simulink model "phdMain"  (R2023b)
settings: Solver=ode4  StartTime=0.0  StopTime=t.Data(end)  FixedStep=1e-3  RelTol=1e-3
undefined symbols (not defined in the file): A_bar, AEFF, B_E, C_bar, C_T, Cd_neg, Cd_pos, DiscIntNeverNeededParam, Gamma, H, k, K, L_gain, L_STROKE, M, m3PsToLpm, P_return_Pa, P_supply_Pa, PA_Pa, PaToBar, PB_Pa, Q, R, RHO, Ts, V01, V02, V_DEAD, v_mPs, W, xc_dot, xc_m
libraries: simulink x1
(part 3 of 3)

== matlab function phdMain/Nguyen Observer/Nguyen_Observer/phi_calc/MATLAB Function4 ==
  data: v input; F_stribeck output
function F_stribeck = fcn(v)


% close all 

% --- Geçiş Yumuşaklığı Parametresi ---
% Bu değer büyüdükçe 0'daki eğim azalır (daha eğimli geçer)
eps_smooth = 0.0223;
% eps_smooth = 0.015;

%%%
kv_p = 12; Fc_p = 25; Fs_p  = 383; tau_p = 0.016;
kv_n = 35; Fc_n = 7.5; Fs_n = 183; tau_n = 0.02016;
%%%


% Yumuşatılmış yön fonksiyonu (sign yerine tanh)
% Bu fonksiyon -1 ile 1 arasında yumuşak bir geçiş sağlar
smooth_sign = tanh(v ./ eps_smooth);

% Asimetrik katsayı vektörleri oluşturma
% Hızın yönüne göre katsayıları seçiyoruz
kv = (v >= 0)*kv_p + (v < 0)*kv_n;
Fc = (v >= 0)*Fc_p + (v < 0)*Fc_n;
Fs = (v >= 0)*Fs_p + (v < 0)*Fs_n;
tau = (v >= 0)*tau_p + (v < 0)*tau_n;
F_stribeck = (Fc .* smooth_sign) + (Fs .* smooth_sign .* exp(-abs(v./tau)));

== matlab function phdMain/SDRE_OBS_SNR/Subsystem/MATLAB Function1 ==
  data: Q1_calc input; Q2_calc input; x1_hat input; B_x output
function B_x = B_x(Q1_calc, Q2_calc, x1_hat)
D_PISTON    = 34e-3;                    % Piston Diameter m
D_ROD       = 30e-3;                    % Rod Diameter m
A_PISTON    = (pi * D_PISTON^2)/4;      % Piston area m^2
A_ROD       = (pi * D_ROD^2)/4;         % Rod area m^2
AEFF        = A_PISTON - A_ROD;         % Effective Area m2
L_STROKE    = 190.16e-3;                % Total Stroke Length m
V01         = AEFF * (L_STROKE/2);      % Initial Chamber Volume in neural position m^3
V02         = AEFF * (L_STROKE/2);      % Initial Chamber Volume in neural position m^3
V_DEAD      = 1.5315e-05;               % 15.3 cm^3 dead volume <- 
V0 = V01 + V_DEAD;                      % Total Volume m3

eps = 1e-6;                             % Epsilon for numerical stability 
%%
A_c = AEFF; 
V_0 = V0; 
beta = 1.6e9; 
%%

delta_1 = beta / ((V_0 + A_c*x1_hat ));
delta_2 = beta / ((V_0 - A_c*x1_hat ));


B_x =   [0; 
             0;
             delta_1 * Q1_calc;
             delta_2 * Q2_calc];% u>=0 ise,

end

== matlab function phdMain/SDRE_OBS_SNR/Subsystem/MATLAB Function2 ==
  data: u input; Q1 output; Ps input; Pr input; x3_hat input; x4_hat input; Q2 output; QR output
function [Q1, Q2, QR] = Q_fcn(u, Ps, Pr, x3_hat, x4_hat)

K_sv           = 0.00000334; 
k_sv           = 1.82709080;
    % x0 parametresini girişten kaldırdık, içeride asimetrik tanımlayacağız.
    
    % --- ASİMETRİK SIZINTI AYARLARI ---
    % Hedef: P_null = 70 bar (Ps=210 bar iken)
    % Bu dengeyi sağlamak için Return tarafı açıklığı daha büyük olmalı.

    % --- GÜNCELLENMİŞ ASİMETRİK SIZINTI AYARLARI ---
    % Hedef: Ps=200 bar, Pr=4.5 bar iken yaklaşık 70-75 bar denge basıncı
    % $$x_{0S} \cdot \sqrt{130} = x_{0R} \cdot \sqrt{70}$$ --> Ortalamaları
    % da bulunan x0 olacak.

    % Ortalama x0 = 0.53e-3 idi. Bunu asimetrik dağıtıyoruz:
    % x0_S = 0.47e-3;  % Supply tarafı (0.47 mA)
    % x0_R = 0.64e-3;  % Return tarafı (0.64 mA)
    
    x0_S = 0.46e-3 ;  % Supply tarafı (0.46 mA) --> bunu editledim
    x0_R = 0.64e-3 ;  % Return tarafı (0.64 mA)

    % x0_S = 0.53e-3;  % Supply tarafı (0.47 mA)
    % x0_R = 0.53e-3;  % Return tarafı (0.64 mA)

    K_tare = 2.345e-9; 
    
    % Güvenlik (Basınçlar)
    dPs1 = max(0, Ps - x3_hat); dP1r = max(0, x3_hat - Pr);
    dPs2 = max(0, Ps - x4_hat); dP2r = max(0, x4_hat - Pr);
    dPsr = max(0, Ps - Pr);

    if u >= 0
        % P_S -> P_1 (Supply Side - Ana Akış) -> x0_S kullan
        Q1_S = K_sv * sqrt(dPs1) * (x0_S + u); 
        
        % P_1 -> P_R (Return Side - Sızıntı) -> x0_R kullan
        Q1_R = K_sv * sqrt(dP1r) * (x0_R^2 / (x0_R + k_sv*u)); 

        % P_S -> P_2 (Supply Side - Sızıntı) -> x0_S kullan
        Q2_S = K_sv * sqrt(dPs2) * (x0_S^2 / (x0_S + k_sv*u)); 
        
        % P_2 -> P_R (Return Side - Ana Akış) -> x0_R kullan
        Q2_R = K_sv * sqrt(dP2r) * (x0_R + u);
    else
        % x < 0 durumu
        % Simetriyi korumak için x negatifken de Supply/Return rollerine göre
        % doğru x0'ı seçmeliyiz.
        
        % P_S -> P_1 (Supply Side - Sızıntı)
        Q1_S = K_sv * sqrt(dPs1) * (x0_S^2 / (x0_S - k_sv*u)); 
        
        % P_1 -> P_R (Return Side - Ana Akış)
        Q1_R = K_sv * sqrt(dP1r) * (x0_R - u); 

        % P_S -> P_2 (Supply Side - Ana Akış)
        Q2_S = K_sv * sqrt(dPs2) * (x0_S - u); 
        
        % P_2 -> P_R (Return Side - Sızıntı)
        Q2_R = K_sv * sqrt(dP2r) * (x0_R^2 / (x0_R - k_sv*u)); 
    end

    Q1 = Q1_S - Q1_R;
    Q2 = Q2_S - Q2_R;
    QR = Q1_R + (Q2_R) + K_tare * sqrt(dPsr); 
end

== matlab function phdMain/SDRE_Observer ==
  settings: updateMethod=DISCRETE  sampleTime=1e-3
  data: u_k input; dxhat output; z_k input; Ps input; Pr input; x_hat input; dP_flat output; P_flat input; x_hat_out output
function [dxhat, dP_flat, x_hat_out] = sdre_observer_ode(u_k, z_k, Ps, Pr, x_hat, P_flat)
% Port sırası:
%   Girişler:  1:u_k(1)  2:z_k(3)  3:Ps(1)  4:Pr(1)  5:x_hat(4)  6:P_flat(16)
%   Çıkışlar:  1:dxhat(4)  2:dP_flat(16)  3:x_hat_out(4)
%
% Integrator 1 → x_hat  (4×1),  IC = [0;0;0;0]
% Integrator 2 → P_flat (16×1), IC = P0(:)  where P0=diag([1e-4,1,1e5,1e5])

    %% Boyut zorlama
    x_hat  = x_hat(:);    % 4×1
    P_flat = P_flat(:);   % 16×1
    z_k    = z_k(:);      % 3×1

    %% Sistem Parametreleri
    m_p    = 3.4;
    D_P    = 34e-3;  D_R = 30e-3;
    A_c    = pi * (D_P^2 - D_R^2) / 4;
    L_S    = 190.16e-3;
    V_DEAD = 1.5315e-5;
    V_0    = A_c * (L_S / 2) + V_DEAD;
    C_t    = 3.9933e-13;
    beta   = 1.6e9;
    K_sv   = 3.34e-6;
    k_sv   = 1.82709080;

    %% Gözlemci Matrisleri
    Q_proc = diag([1e-3, 1e-2, 5e8, 5e8]);
    R_inv  = diag([1.0e7, 1.0e-2, 1.0e-2]);
    H      = [1 0 0 0;
              0 0 1 0;
              0 0 0 1];

    %% P matrisini yeniden oluştur
    P  = reshape(P_flat, 4, 4);

    x1 = x_hat(1);  x2 = x_hat(2);
    x3 = x_hat(3);  x4 = x_hat(4);

    %% Durum Bağımlı Matrisler
    A_k = local_A(x1, x2, beta, V_0, A_c, C_t, m_p);
    [Q1, Q2] = local_Q(u_k, Ps, Pr, x3, x4, K_sv, k_sv);
    f_k = local_B(x1, beta, V_0, A_c, Q1, Q2);

    %% Kalman Kazancı
    PHt = P * H';
    K   = PHt * R_inv;

    %% Gözlemci türevi
    dxhat = A_k * x_hat + f_k + K * (z_k - H * x_hat);

    %% Diferansiyel Riccati
    dP      = A_k*P + P*A_k' - PHt*R_inv*(H*P) + Q_proc;
    dP_flat = dP(:);

    x_hat_out = x_hat;
end

%% ---- Yerel Fonksiyonlar ----
function A_x = local_A(x1, x2, beta, V0, Ac, Ct, m)
    eps_v = 1e-6;
    if x2 >= 0
        Fc=6.93;   Fs=93.02;  tau_f=0.0357;  B=33.96;
    else
        Fc=19.39;  Fs=83.58;  tau_f=0.0382;  B=31.98;
    end
    Ff = tanh(x2)*(Fc + (Fs-Fc)*exp(-abs(x2)/tau_f));
    d1 = beta/(V0 + Ac*x1);
    d2 = beta/(V0 - Ac*x1);
    A_x = [0   1                             0        0    ;
           0  -B/m - Ff/(m*abs(x2)+eps_v)   Ac/m    -Ac/m ;
           0  -d1*Ac                        -d1*Ct    d1*Ct;
           0   d2*Ac                         d2*Ct   -d2*Ct];
end

function [Q1, Q2] = local_Q(x, Ps, Pr, P1, P2, K, k)
    x0S=0.46e-3;  x0R=0.64e-3;
    dPs1=max(0.0,Ps-P1);  dP1r=max(0.0,P1-Pr);
    dPs2=max(0.0,Ps-P2);  dP2r=max(0.0,P2-Pr);
    if x >= 0
        Q1 = K*sqrt(dPs1)*(x0S+x)           - K*sqrt(dP1r)*(x0R^2/(x0R+k*x));
        Q2 = K*sqrt(dPs2)*(x0S^2/(x0S+k*x)) - K*sqrt(dP2r)*(x0R+x);
    else
        Q1 = K*sqrt(dPs1)*(x0S^2/(x0S-k*x)) - K*sqrt(dP1r)*(x0R-x);
        Q2 = K*sqrt(dPs2)*(x0S-x)            - K*sqrt(dP2r)*(x0R^2/(x0R-k*x));
    end
end

function Bv = local_B(x1, beta, V0, Ac, Q1, Q2)
    Vd = 1.5315e-5;
    d1 = beta/(V0+Ac*x1+Vd);
    d2 = beta/(V0-Ac*x1+Vd);
    Bv = [0; 0; d1*Q1; d2*Q2];
end

== matlab function phdMain/SDRE_OBS_SNR/MATLAB Function3 ==
  data: x_1_hat input; A_k output; x_2_hat input
function A_k = A_k_discrete(x_1_hat, x_2_hat)
M           = 3.4;                      % Movable mass (Piston + Rod) kg
D_PISTON    = 34e-3;                    % Piston Diameter m
D_ROD       = 30e-3;                    % Rod Diameter m
A_PISTON    = (pi * D_PISTON^2)/4;      % Piston area m^2
A_ROD       = (pi * D_ROD^2)/4;         % Rod area m^2
AEFF        = A_PISTON - A_ROD;         % Effective Area m2
L_STROKE    = 190.16e-3;                % Total Stroke Length m
V01         = AEFF * (L_STROKE/2);      % Initial Chamber Volume in neural position m^3
V02         = AEFF * (L_STROKE/2);      % Initial Chamber Volume in neural position m^3
V_DEAD      = 1.5315e-05;               % 15.3 cm^3 dead volume 
V0          = V01 + V_DEAD;             % Total Volume m3
C_T         = 3.9933e-13;               % Internal leakage constant m3/s/Pa
eps_val     = 1e-6;                     % Epsilon for numerical stability 

%% Parametre Atamaları
m = M; 
C_t = C_T; 
A_c = AEFF; 
V_0 = V0; 
beta = 1.6e9; 
Ts = 1e-3; 
%% Sürtünme Dinamikleri ve Sönüm Katsayısı
if x_2_hat >= 0 
    F_c = 6.93; 
    F_s = 93.02; 
    tau = 0.0357; 
    B = 33.96; 
else 
    F_c = 19.39; 
    F_s = 83.58; 
    tau = 0.0382; 
    B = 31.98; 
end 

% Sürtünme denkleminde sign yerine tanh kullanımı (Sürekli türevlenebilirlik için)
F_frc = tanh(x_2_hat) * (F_c + (F_s - F_c) * exp(-abs(x_2_hat) / tau)); 

%% Matris Elemanlarının Hesaplanması (Sürekli Zaman Ac)
delta_1 = beta / (V_0 + A_c * x_1_hat);
delta_2 = beta / (V_0 - A_c * x_1_hat);

a22 = -B/m - F_frc / (m * abs(x_2_hat) + eps_val);
a23 = A_c/m;
a24 = -A_c/m;
a32 = -delta_1 * A_c; 
a33 = -delta_1 * C_t;
a34 = delta_1 * C_t;
a42 = delta_2 * A_c;
a43 = delta_2 * C_t;
a44 = -delta_2 * C_t;

% Sürekli Zaman Durum Matrisi
A_c_mat = [0    1       0       0; 
           0    a22     a23     a24; 
           0    a32     a33     a34; 
           0    a42     a43     a44];

%% Tustin Yöntemi ile Ayrıklaştırma (Discrete Time Ak)
I = eye(4);
% (I - 0.5*Ts*Ac)^-1 * (I + 0.5*Ts*Ac) işlemi sayısal verimlilik için mldivide (\) ile çözülür
A_k = (I - 0.5 * Ts * A_c_mat) \ (I + 0.5 * Ts * A_c_mat);

end

== matlab function phdMain/SDRE_OBS_SNR/MATLAB Function4 ==
  data: Q1_calc input; Q2_calc input; x1_hat input; B_k output; A_k input
function B_k = B_k_discrete(Q1_calc, Q2_calc, x1_hat, A_k)
    % Fiziksel Parametreler
    D_PISTON    = 34e-3;                    % Piston Diameter m
    D_ROD       = 30e-3;                    % Rod Diameter m
    A_PISTON    = (pi * D_PISTON^2)/4;      % Piston area m^2
    A_ROD       = (pi * D_ROD^2)/4;         % Rod area m^2
    AEFF        = A_PISTON - A_ROD;         % Effective Area m2
    L_STROKE    = 190.16e-3;                % Total Stroke Length m
    V01         = AEFF * (L_STROKE/2);      % Initial Chamber Volume m^3
    V_DEAD      = 1.5315e-05;               % 15.3 cm^3 dead volume 
    V0          = V01 + V_DEAD;             % Total Volume m3
    
    A_eff_area  = AEFF; 
    beta        = 1.6e9; 
    Ts = 1e-3; 
    
    % Sürekli Zaman B_c Vektörünün Hesaplanması
    delta_1 = beta / (V0 + A_eff_area * x1_hat);
    delta_2 = beta / (V0 - A_eff_area * x1_hat);
    
    B_c = [0; 
           0;
           delta_1 * Q1_calc;
           delta_2 * Q2_calc];
           
    % Tustin cebirsel dönüşümü ile Ak entegrasyonu
    I = eye(4);
    B_k = (Ts / 2) * (I + A_k) * B_c;
end

== matlab function phdMain/SDRE_OBS_SNR/MATLAB Function5 ==
  data: x_hat input; A_k output; u_k input; B_k output; Ps_k input; Pr_k input
function [A_k, B_k] = discrete_system_matrices(x_hat, u_k, Ps_k, Pr_k)
    % 1. Sistem Geometrisi ve Tanımlamalar
    x1_hat = x_hat(1); 
    x2_hat = x_hat(2); 
    x3_hat = x_hat(3); 
    x4_hat = x_hat(4); 
    
    M           = 3.4;
    D_PISTON    = 34e-3;
    D_ROD       = 30e-3;
    A_eff_area  = (pi * D_PISTON^2)/4 - (pi * D_ROD^2)/4;
    L_STROKE    = 190.16e-3;
    V0          = A_eff_area * (L_STROKE/2) + 1.5315e-05;
    C_t         = 3.9933e-13;
    eps_val     = 1e-6;
    B_E = 1.6e9;
%%
    % 2. Sürtünme ve Diferansiyel Değişkenler
    if x2_hat >= 0 
        F_c = 6.93; F_s = 93.02; tau = 0.0357; B = 33.96; 
    else 
        F_c = 19.39; F_s = 83.58; tau = 0.0382; B = 31.98; 
    end 

    F_frc = tanh(x2_hat) * (F_c + (F_s - F_c) * exp(-(abs(x2_hat)^2) / tau^2)); 
    
    delta_1 = B_E / (V0 + A_eff_area * x1_hat + eps_val);
    delta_2 = B_E / (V0 - A_eff_area * x1_hat + eps_val);

    % 3. Sürekli Zaman Ac Matris Elemanları
    a22 = -B/M - F_frc / ((M * x2_hat) + eps_val);

    a23 = A_eff_area/M;  a24 = -A_eff_area/M;
    a32 = -delta_1 * A_eff_area; 
    a33 = -delta_1 * C_t; 
    a34 = delta_1 * C_t;
    a42 = delta_2 * A_eff_area;  
    a43 = delta_2 * C_t;  
    a44 = -delta_2 * C_t;

    A_c_mat = [0    1       0       0; 
               0    a22     a23     a24; 
               0    a32     a33     a34; 
               0    a42     a43     a44];
    

      % Valf Parametreleri
    K_sv = 0.00000334; 
    k_sv = 1.82709080;
    K_tare = 2.345e-9; 
    
    % Asimetrik Sızıntı Ayarları (Sıfır Geçiş Dengesi)
    x0_S = 0.46e-3;  % Supply tarafı (0.46 mA)
    x0_R = 0.64e-3;  % Return tarafı (0.64 mA)
    
    % Basınç Düşümleri (Kareköklü ifadelerde karmaşık sayıları önlemek için max(0,.) kullanımı)
    dPs1 = max(0, Ps_k - x3_hat); 
    dP1r = max(0, x3_hat - Pr_k);
    dPs2 = max(0, Ps_k - x4_hat); 
    dP2r = max(0, x4_hat - Pr_k);
    dPsr = max(0, Ps_k - Pr_k);

    % Akış Denklemleri
    if u_k >= 0
        % P_S -> P_1 (Supply Side - Ana Akış) 
        Q1_S = K_sv * sqrt(dPs1) * (x0_S + u_k); 
        
        % P_1 -> P_R (Return Side - Sızıntı) 
        Q1_R = K_sv * sqrt(dP1r) * (x0_R^2 / (x0_R + k_sv * u_k)); 
        
        % P_S -> P_2 (Supply Side - Sızıntı) 
        Q2_S = K_sv * sqrt(dPs2) * (x0_S^2 / (x0_S + k_sv * u_k)); 
        
        % P_2 -> P_R (Return Side - Ana Akış) 
        Q2_R = K_sv * sqrt(dP2r) * (x0_R + u_k);
    else
        % u_k < 0 Durumu
        % P_S -> P_1 (Supply Side - Sızıntı)
        Q1_S = K_sv * sqrt(dPs1) * (x0_S^2 / (x0_S - k_sv * u_k)); 
        
        % P_1 -> P_R (Return Side - Ana Akış)
        Q1_R = K_sv * sqrt(dP1r) * (x0_R - u_k); 
        
        % P_S -> P_2 (Supply Side - Ana Akış)
        Q2_S = K_sv * sqrt(dPs2) * (x0_S - u_k); 
        
        % P_2 -> P_R (Return Side - Sızıntı)
        Q2_R = K_sv * sqrt(dP2r) * (x0_R^2 / (x0_R - k_sv * u_k)); 
    end

    % Net Odacık Akışları ve Dönüş Akışı
    Q1 = Q1_S - Q1_R;
    Q2 = Q2_S - Q2_R;
    QR = Q1_R + Q2_R + K_tare * sqrt(dPsr); 

    % 4. Sürekli Zaman Bc Vektör Elemanları
    B_c_vec = [0; 0; delta_1 * Q1; delta_2 * Q2];

    % 5. Tustin Ayrıklaştırma ve Karşılıklı Entegrasyon
    I = eye(4);

    A_k = A_c_mat; % (I - A_c_mat) \ (I + 0.5 * Ts * A_c_mat); % 0.5 * Ts
    B_k = B_c_vec; % (I + A_k) * B_c_vec; % (Ts / 2) * 
end

== matlab function phdMain/SDRE_Observer1 ==
  settings: updateMethod=DISCRETE  sampleTime=1e-3
  data: u_k input; x_hat_out output; z_k input; Ps input; Pr input
function x_hat_out = sdre_observer(u_k, z_k, Ps, Pr)
%SDRE_OBSERVER  Discrete-time SDRE Observer, Ts=1e-3s
% u_k: valf [m](1x1), z_k:[xc;P1;P2][m,Pa,Pa](3x1), Ps,Pr:[Pa](1x1)
% x_hat_out: [x_c;v_c;P1;P2] (4x1)
    coder.extrinsic('care','eig');
    dt=1e-3; m=3.4;
    D_P=34e-3; D_R=30e-3;
    A_c=pi*(D_P^2-D_R^2)/4;
    L_S=190.16e-3; V_DEAD=1.5315e-5;
    V_0=A_c*(L_S/2)+V_DEAD;
    C_t=3.9933e-13; beta=1.6e9;
    K_sv=3.34e-6; k_sv=1.82709080;
    Q_proc=diag([1e-3,1e-2,5e8,5e8]);
    R_meas=diag([1e-7,1e2,1e2]);
    H=[1 0 0 0; 0 0 1 0; 0 0 0 1];
    SC=[1;1;1e-7;1e-7]; SC_INV=[1;1;1e7;1e7];
    persistent x_hat P_k;
    if isempty(x_hat)
        x_hat=[0;0;z_k(2);z_k(3)];
        P_k=diag([1e-4,1,1e5,1e5]);
    end
    x1=x_hat(1); x2=x_hat(2); x3=x_hat(3); x4=x_hat(4);
    A_k=local_A(x1,x2,beta,V_0,A_c,C_t,m);
    [Q1,Q2]=local_Q(u_k,Ps,Pr,x3,x4,K_sv,k_sv);
    B_k=local_B(x1,beta,V_0,A_c,Q1,Q2);
    P_new=zeros(4,4);
    P_new=care(A_k',H',Q_proc,R_meas);
    ev=zeros(4,1); ev=eig(P_new);
    if isreal(P_new)&&all(ev>-1e-6), P_k=P_new; end
    K_k=(R_meas\(H*P_k))';
    I4=eye(4);
    A_cl=A_k-K_k*H; U_cl=B_k+K_k*z_k;
    A_sc=(SC*SC_INV').*A_cl;
    x_sc=SC.*x_hat; U_sc=SC.*U_cl;
    LHS=I4-0.5*dt*A_sc;
    RHS=(I4+0.5*dt*A_sc)*x_sc+dt*U_sc;
    x_hat=SC_INV.*(LHS\RHS);
    x_hat_out=x_hat;
end
function A_x=local_A(x1,x2,beta,V0,Ac,Ct,m)
    eps_v=1e-6;
    if x2>=0, Fc=6.93; Fs=93.02; tau_f=0.0357; B=33.96;
    else,     Fc=19.39;Fs=83.58; tau_f=0.0382; B=31.98; end
    Ff=tanh(x2)*(Fc+(Fs-Fc)*exp(-abs(x2)/tau_f));
    d1=beta/(V0+Ac*x1); d2=beta/(V0-Ac*x1);
    A_x=[0  1                        0      0   ;
         0 -B/m-Ff/(m*abs(x2)+eps_v) Ac/m  -Ac/m;
         0 -d1*Ac                   -d1*Ct  d1*Ct;
         0  d2*Ac                    d2*Ct -d2*Ct];
end
function [Q1,Q2]=local_Q(x,Ps,Pr,P1,P2,K,k)
    x0S=0.46e-3; x0R=0.64e-3;
    dPs1=max(0,Ps-P1); dP1r=max(0,P1-Pr);
    dPs2=max(0,Ps-P2); dP2r=max(0,P2-Pr);
    if x>=0
        Q1=K*sqrt(dPs1)*(x0S+x)         -K*sqrt(dP1r)*(x0R^2/(x0R+k*x));
        Q2=K*sqrt(dPs2)*(x0S^2/(x0S+k*x))-K*sqrt(dP2r)*(x0R+x);
    else
        Q1=K*sqrt(dPs1)*(x0S^2/(x0S-k*x))-K*sqrt(dP1r)*(x0R-x);
        Q2=K*sqrt(dPs2)*(x0S-x)           -K*sqrt(dP2r)*(x0R^2/(x0R-k*x));
    end
end
function Bv=local_B(x1,beta,V0,Ac,Q1,Q2)
    Vd=1.5315e-5;
    d1=beta/(V0+Ac*x1+Vd); d2=beta/(V0-Ac*x1+Vd);
    Bv=[0;0;d1*Q1;d2*Q2];
end

== matlab function phdMain/SDRE_OBS_SNR/MATLAB Function1 ==
  data: u_k input; x_hat_dot output; y_k input; A_k input; B_k input; P_plus output; H input; Q input; R input; x_hat_prev input; P_prev input; K_k output
function [x_hat_dot, P_plus, K_k] = discrete_sdre_kf(u_k, y_k, A_k, B_k, H, Q, R, x_hat_prev, P_prev)
    % discrete_sdre_kf: Ayrık Zaman Durum Bağımlı Kalman Filtresi
    % 
    % Girdiler:
    % u_k        : k anındaki kontrol girişi
    % y_k        : k anındaki sensör ölçüm vektörü
    % A_k, B_k   : Tustin ile ayrıklaştırılmış anlık sistem matrisleri
    % H          : Gözlem matrisi (Görsellerdeki C_k)
    % Q, R       : Süreç ve ölçüm gürültüsü kovaryans matrisleri
    % x_hat_prev : k-1 anındaki güncellenmiş durum tahmini (x_hat_plus_{k-1})
    % P_prev     : k-1 anındaki güncellenmiş hata kovaryansı (P_plus_{k-1})
    %
    % Çıktılar:
    % x_hat_plus : k anındaki a posteriori durum tahmini
    % P_plus     : k anındaki a posteriori hata kovaryans matrisi
    % K_k        : k anındaki Kalman kazancı

    %% 1. ZAMAN GÜNCELLEMESİ (PREDICTION / TAHMİN ADIMI)
    % A priori (öncül) durum ve kovaryans tahminleri
    x_hat = A_k * x_hat_prev + B_k; % Debiler u ile hesaplandığı için tekrar çarpılmadı.
    P_minus     = A_k * P_prev * A_k' + Q;
    
    %% 2. KAZANÇ HESABI (KALMAN GAIN)
    % İnovasyon (Artık) Kovaryansı
    S_k = H * P_minus * H' + R;
    
    % Kalman Kazancı
    % Matematiksel karşılık: K_k = P_minus * H^T * S_k^-1
    % Sayısal verimlilik ve kararlılık için ters alma (inv) yerine lineer denklem çözücü (\) kullanılır:
    % K_k = (S_k \ (H * P_minus)')'; 
    K_k = (P_minus * H') / S_k;
    %% 3. ÖLÇÜM GÜNCELLEMESİ (CORRECTION / DÜZELTME ADIMI)
    % A posteriori (sonsıl) durum tahmini
    x_hat_dot = x_hat + K_k * (y_k - H * x_hat);
    
    % A posteriori hata kovaryans matrisi
    I = eye(size(A_k));
    P_plus = (I - K_k * H) * P_minus;
    
    % Kovaryans matrisinin simetrikliğinin korunması (Sayısal yuvarlama hatalarına karşı önlem)
    P_plus = (P_plus + P_plus') / 2;
end

== matlab function phdMain/SDRE_Observer2 ==
  settings: updateMethod=DISCRETE  sampleTime=1e-3
  data: u_k input; x_hat_out output; z_k input; Ps input; Pr input
function x_hat_out = sdre_observer_discrete(u_k, z_k, Ps, Pr)
%SDRE_OBSERVER_DISCRETE  NI CompactRIO — 1 kHz
%
% Kod üretimi uyumlu: care / eig / extrinsic YOK
% Her adımda K Riccati rekürasyonuyla güncellenir
%
% Girişler:
%   u_k  (1×1) : valf komutu [m]
%   z_k  (3×1) : [x_c (m); P1 (Pa); P2 (Pa)]
%   Ps   (1×1) : besleme basıncı [Pa]
%   Pr   (1×1) : dönüş basıncı  [Pa]
%
% Çıkış:
%   x_hat_out (4×1) : [x_c; v_c; P1; P2]
%
% Sample time : 1e-3 s  (bloğa atayın)

    %% Kalıcı durum (kod üretiminde static değişkene dönüşür)
    persistent x_hat P_k;
    if isempty(x_hat)
        x_hat = zeros(4,1);
        P_k   = diag([1e-4, 1, 1e5, 1e5]);
    end

    %% Sistem parametreleri
    dt     = 1e-3;
    m_p    = 3.4;
    D_P    = 34e-3;    D_R = 30e-3;
    A_c    = pi*(D_P^2 - D_R^2)/4;
    L_S    = 190.16e-3;
    V_DEAD = 1.5315e-5;
    V_0    = A_c*(L_S/2) + V_DEAD;
    C_t    = 3.9933e-13;
    beta   = 1.6e9;
    K_sv   = 3.34e-6;
    k_sv   = 1.82709080;

    %% Gözlemci matrisleri
    % Q_d = dt * Q_sürekli — ayrık süreç gürültüsü
    Q_d    = diag([1e-6, 1e-5, 5e5, 5e5]);
    R_meas = diag([1e-7, 1e2,  1e2]);
    H      = [1 0 0 0;
              0 0 1 0;
              0 0 0 1];
    I4     = eye(4);

    %% Ölçekleme (trapezoidal adım için RCOND koruması)
    SC     = [1; 1; 1e-7; 1e-7];
    SC_INV = [1; 1; 1e7;  1e7 ];

    %% Mevcut durum
    z_k = z_k(:);
    x1 = x_hat(1);  x2 = x_hat(2);
    x3 = x_hat(3);  x4 = x_hat(4);

    %% Durum bağımlı matrisler A(x), f(x,u)
    A_k = local_A(x1, x2, beta, V_0, A_c, C_t, m_p);
    [Q1, Q2] = local_Q(u_k, Ps, Pr, x3, x4, K_sv, k_sv);
    f_k = local_B(x1, beta, V_0, A_c, Q1, Q2);

    %% ============================================================
    %%  RİCCATİ REKÜRASYONU (her adımda K güncellenir)
    %% ============================================================

    % 1. Öngörü: A_d = I + dt*A_k  (Euler ayrıklaştırma)
    A_d    = I4 + dt * A_k;
    P_pred = A_d * P_k * A_d' + Q_d;      % 4×4

    % 2. Yenilik kovaryansı S  (yalnızca 3×3 — verimli)
    S = H * P_pred * H' + R_meas;          % 3×3

    % 3. Kalman kazancı: K = P_pred * H' / S
    K_k = (P_pred * H') / S;               % 4×3

    % 4. Kovaryans güncelleme — Joseph formu
    %    (simetri + pozitif kesinlik garanti altında)
    IKH = I4 - K_k * H;
    P_k = IKH * P_pred * IKH' + K_k * R_meas * K_k';   % 4×4

    %% ============================================================
    %%  DURUM GÜNCELLEMESİ — Trapezoidal + ölçekleme
    %% ============================================================
    A_cl = A_k - K_k * H;
    U_cl = f_k + K_k * z_k;

    A_sc  = (SC * SC_INV') .* A_cl;
    x_sc  = SC .* x_hat;
    U_sc  = SC .* U_cl;
    LHS   = I4 - 0.5*dt*A_sc;
    RHS   = (I4 + 0.5*dt*A_sc)*x_sc + dt*U_sc;
    x_hat = SC_INV .* (LHS \ RHS);

    x_hat_out = x_hat;
end

%% ======================================================
%%  YEREL FONKSİYONLAR
%% ======================================================

function A_x = local_A(x1, x2, beta, V0, Ac, Ct, m)
    eps_v = 1e-6;
    if x2 >= 0
        Fc=6.93;   Fs=93.02;  tau_f=0.0357;  B=33.96;
    else
        Fc=19.39;  Fs=83.58;  tau_f=0.0382;  B=31.98;
    end
    Ff = tanh(x2)*(Fc + (Fs-Fc)*exp(-abs(x2)/tau_f));
    d1 = beta/(V0 + Ac*x1);
    d2 = beta/(V0 - Ac*x1);
    A_x = [0   1                             0        0    ;
           0  -B/m - Ff/(m*abs(x2)+eps_v)   Ac/m    -Ac/m ;
           0  -d1*Ac                        -d1*Ct    d1*Ct;
           0   d2*Ac                         d2*Ct   -d2*Ct];
end

function [Q1, Q2] = local_Q(x, Ps, Pr, P1, P2, K, k)
    x0S=0.46e-3;  x0R=0.64e-3;
    dPs1=max(0.0,Ps-P1);  dP1r=max(0.0,P1-Pr);
    dPs2=max(0.0,Ps-P2);  dP2r=max(0.0,P2-Pr);
    if x >= 0
        Q1 = K*sqrt(dPs1)*(x0S+x)           - K*sqrt(dP1r)*(x0R^2/(x0R+k*x));
        Q2 = K*sqrt(dPs2)*(x0S^2/(x0S+k*x)) - K*sqrt(dP2r)*(x0R+x);
    else
        Q1 = K*sqrt(dPs1)*(x0S^2/(x0S-k*x)) - K*sqrt(dP1r)*(x0R-x);
        Q2 = K*sqrt(dPs2)*(x0S-x)            - K*sqrt(dP2r)*(x0R^2/(x0R-k*x));
    end
end

function Bv = local_B(x1, beta, V0, Ac, Q1, Q2)
    Vd=1.5315e-5;
    d1=beta/(V0+Ac*x1+Vd);
    d2=beta/(V0-Ac*x1+Vd);
    Bv=[0; 0; d1*Q1; d2*Q2];
end

== matlab function phdMain/old/MATLAB Function2 ==
  data: xv input; Q1 output; P_P input; P_T input; P_A input; P_B input; Q2 output; Q_RETURN output
function [Q1, Q2, Q_RETURN] = fcn_Valve_Tamburrano_Hybrid( ...
    xv, P_P, P_T, P_A, P_B)

% SI units:
% xv [m], P_* [Pa], w,c,r [m], rho [kg/m^3], mu [Pa*s], Cd [-]
%
% Outputs:
%   Q_A, Q_B         : Port net flows [m^3/s]
%   Q_Leak_Total     : leakage indicator [m^3/s]
%   Q_return_lpm     : total return flow to return line [LPM]

%% 0) Checks

%%
k = 0.2; 
K = 1.7817e-6; 
x0 = 0.00099959586;

x = xv;
P_S = P_P;
P_A = P_A; 
P_B = P_B;
P_R = P_T;

K1_S = K;
K1_R = K; 
K2_S = K; 
K2_R = K; 

k1_s = k; 
k1_r = k; 
k2_s = k; 
k2_r = k; 

%% 
if x >= 0
        % For control port 1
        Q1_S = K1_S * sqrt(abs(P_S - P_A)) * (x0 + x) * sign(P_S - P_A);
        Q1_R = K1_R * sqrt(abs(P_A - P_R)) * (x0^2) * ((x0 + k1_r*x)^-1) *sign(P_A - P_R);

        % For control port 2
        Q2_S = K2_S * sqrt(abs(P_S - P_B)) * (x0^2) * ((x0 + k2_s*x)^-1) *sign((P_S - P_B)); 
        Q2_R = K2_R * sqrt(abs(P_B - P_R)) * (x0 + x) * sign((P_B - P_R)); 
else 
        % For control port 1
        Q1_S = K1_S * sqrt(abs(P_S - P_A)) * (x0^2) * ((x0 - k1_s*x)^-1) * sign(P_S - P_A);
        Q1_R = K1_R * sqrt(abs(P_A - P_R)) * (x0 - x) * sign(P_A - P_R);

        % For control port 2
        Q2_S = K2_S * sqrt(abs(P_S - P_B)) * (x0 - x) * sign(P_S - P_B); 
        Q2_R = K2_R * sqrt(abs(P_B - P_R)) * (x0^2) * ((x0 - k2_r*x)^-1)* sign(P_B - P_R); 
end 

Q1 = Q1_S - Q1_R; 
Q2 = Q2_S - Q2_R; 

Q_RETURN = Q1_R + Q2_R;

== matlab function phdMain/Subsystem1/MATLAB Function ==
  data: Q1 output; Q2 output; x input; Ps input; Pr input; P1 input; P2 input; K input; k input; QR output
function [Q1, Q2, QR] = fcn(x, Ps, Pr, P1, P2, K, k)
    % x0 parametresini girişten kaldırdık, içeride asimetrik tanımlayacağız.
    
    % --- ASİMETRİK SIZINTI AYARLARI ---
    % Hedef: P_null = 70 bar (Ps=210 bar iken)
    % Bu dengeyi sağlamak için Return tarafı açıklığı daha büyük olmalı.

    % --- GÜNCELLENMİŞ ASİMETRİK SIZINTI AYARLARI ---
    % Hedef: Ps=200 bar, Pr=4.5 bar iken yaklaşık 70-75 bar denge basıncı
    % $$x_{0S} \cdot \sqrt{130} = x_{0R} \cdot \sqrt{70}$$ --> Ortalamaları
    % da bulunan x0 olacak.

    % Ortalama x0 = 0.53e-3 idi. Bunu asimetrik dağıtıyoruz:
    % x0_S = 0.47e-3;  % Supply tarafı (0.47 mA)
    % x0_R = 0.64e-3;  % Return tarafı (0.64 mA)
    
    x0_S = 0.46e-3 ;  % Supply tarafı (0.46 mA) --> bunu editledim
    x0_R = 0.64e-3 ;  % Return tarafı (0.64 mA)

    % x0_S = 0.53e-3;  % Supply tarafı (0.47 mA)
    % x0_R = 0.53e-3;  % Return tarafı (0.64 mA)

    K_tare = 2.345e-9; 
    
    % Güvenlik (Basınçlar)
    dPs1 = max(0, Ps - P1); dP1r = max(0, P1 - Pr);
    dPs2 = max(0, Ps - P2); dP2r = max(0, P2 - Pr);
    dPsr = max(0, Ps - Pr);

    if x >= 0
        % P_S -> P_1 (Supply Side - Ana Akış) -> x0_S kullan
        Q1_S = K * sqrt(dPs1) * (x0_S + x); 
        
        % P_1 -> P_R (Return Side - Sızıntı) -> x0_R kullan
        Q1_R = K * sqrt(dP1r) * (x0_R^2 / (x0_R + k*x)); 

        % P_S -> P_2 (Supply Side - Sızıntı) -> x0_S kullan
        Q2_S = K * sqrt(dPs2) * (x0_S^2 / (x0_S + k*x)); 
        
        % P_2 -> P_R (Return Side - Ana Akış) -> x0_R kullan
        Q2_R = K * sqrt(dP2r) * (x0_R + x);
    else
        % x < 0 durumu
        % Simetriyi korumak için x negatifken de Supply/Return rollerine göre
        % doğru x0'ı seçmeliyiz.
        
        % P_S -> P_1 (Supply Side - Sızıntı)
        Q1_S = K * sqrt(dPs1) * (x0_S^2 / (x0_S - k*x)); 
        
        % P_1 -> P_R (Return Side - Ana Akış)
        Q1_R = K * sqrt(dP1r) * (x0_R - x); 

        % P_S -> P_2 (Supply Side - Ana Akış)
        Q2_S = K * sqrt(dPs2) * (x0_S - x); 
        
        % P_2 -> P_R (Return Side - Sızıntı)
        Q2_R = K * sqrt(dP2r) * (x0_R^2 / (x0_R - k*x)); 
    end

    Q1 = Q1_S - Q1_R;
    Q2 = Q2_S - Q2_R;
    QR = Q1_R + (Q2_R) + K_tare * sqrt(dPsr); 
end

== matlab function phdMain/Cylinder_Dynamics/Subsystem1/MATLAB Function1 ==
  data: x input; F_end output; x_dot input; xmin input; xmax input; k_end input; v_lock input
function F_end = endstop_force_simple(x, x_dot, xmin, xmax, k_end, v_lock)
%#codegen
% Very stable end-stop with velocity locking
% Minimal oscillation, solver-friendly

% v_lock : velocity below which motion is considered zero (m/s)
% Typical: 1e-3 … 5e-3

F_end = 0.0;
ccc = 1e6; 
% ---- LOWER STOP ----
if x <= xmin
    % spring force
    F_end = k_end * (xmin - x);

    % velocity lock (kill oscillation)
    if x_dot < v_lock
        F_end = F_end - ccc * x_dot;   % artificial strong damping
    end
end

% ---- UPPER STOP ----
if x >= xmax
    % spring force
    F_end = -k_end * (x - xmax);

    % velocity lock
    if x_dot > -v_lock
        F_end = F_end - ccc * x_dot;
    end
end

== matlab function phdMain/old/Flow_Calc_WithLeak/MATLAB Function2 ==
  data: xv input; Q_A output; P_P input; P_T input; P_R input; P_A input; P_B input; w input; Q_B output; Q_Leak_Total_lpm output; c input; r input; rho input; mu input; Cd input; bias_P_dynamic input; bias_T_dynamic input; Q_return_model_lpm output; x_leak input
function [Q_A, Q_B, Q_Leak_Total_lpm, Q_return_model_lpm] = fcn_Valve_Tamburrano_Hybrid( ...
    xv, P_P, P_T, P_R, P_A, P_B, w, c, r, rho, mu, Cd, ...
    bias_P_dynamic, bias_T_dynamic, x_leak)

% SI units:
% xv [m], P_* [Pa], w,c,r [m], rho [kg/m^3], mu [Pa*s], Cd [-]
%
% Outputs:
%   Q_A, Q_B         : Port net flows [m^3/s]
%   Q_Leak_Total     : leakage indicator [m^3/s]
%   Q_return_lpm     : total return flow to return line [LPM]

%% 0) Checks
if c <= 0 || w <= 0 || rho <= 0 || mu <= 0 || Cd <= 0 || r < 0
    error('SI parametreler: w>0, c>0, r>=0, rho>0, mu>0, Cd>0 olmalı.');
end

%% 1) Tamburrano Eq.(19) -> l_eff (r,c'den)
if r == 0
    l_eff = c;
else
    y = (-(2*c + 4*r) + sqrt((2*c + 4*r)^2 + 16*r^2)) / 2; % y=l-c
    y = max(y, 0);
    l_eff = c + y;
end

%% 2) Tamburrano Eq.(18): laminer leakage conductance
K_lam_base = (pi * w * (l_eff^2)) / (32 * mu);  % [m^3/(s*Pa)]

%% 3) Static/Dynamic bias (pressure-holding + dynamic offset reduction)
transition_width = 20.5e-5;           % [m] (tune)
move_factor = tanh(abs(xv)/transition_width);

% --- Static
bias_P_static = 0.460;
bias_T_static = 0.9050;

% --- Interpolate to dynamic values ---
leak_bias_P = bias_P_static*(1-move_factor) + bias_P_dynamic*move_factor;
leak_bias_T = bias_T_static*(1-move_factor) + bias_T_dynamic*move_factor;


leak_bias_P = max(leak_bias_P, 0);
leak_bias_T = max(leak_bias_T, 0);



%% 4) Null-weighting for laminar leakage (keeps M-profile in motion)
% x_leak = 2.0e-4;                      % [m] (tune)
g = exp(-(abs(xv)/x_leak)^2);

%% 5) Metering areas
A_open = w * abs(xv);

if xv >= 0
    Area_PA = A_open;  Area_AT = 0;
    Area_PB = 0;       Area_BT = A_open;
else
    Area_PA = 0;       Area_AT = A_open;
    Area_PB = A_open;  Area_BT = 0;
end

%% 6) ΔP
dP_PA = (P_P - P_A);
dP_AT = (P_A - P_T);
dP_PB = (P_P - P_B);
dP_BT = (P_B - P_T);

%% 7) Orifice flows (Eq.7–10)
Q_PA_or = Cd * Area_PA * sign(dP_PA) * sqrt(2/rho * abs(dP_PA));
Q_AT_or = Cd * Area_AT * sign(dP_AT) * sqrt(2/rho * abs(dP_AT));
Q_PB_or = Cd * Area_PB * sign(dP_PB) * sqrt(2/rho * abs(dP_PB));
Q_BT_or = Cd * Area_BT * sign(dP_BT) * sqrt(2/rho * abs(dP_BT));

%% 8) Laminar leakage flows (Eq.18) with bias + null-weighting g
Q_PA_lam = (K_lam_base * leak_bias_P) * dP_PA;
Q_PB_lam = (K_lam_base * leak_bias_P) * dP_PB;
Q_AT_lam = (K_lam_base * leak_bias_T) * dP_AT;
Q_BT_lam = (K_lam_base * leak_bias_T) * dP_BT;

Q_PA = Q_PA_or + g * Q_PA_lam;
Q_PB = Q_PB_or + g * Q_PB_lam;
Q_AT = Q_AT_or + g * Q_AT_lam;
Q_BT = Q_BT_or + g * Q_BT_lam;

%% 9) Port net flows
Q_A = Q_PA - Q_AT;
Q_B = Q_PB - Q_BT;

%% 10) Return-line measured flow (valve-to-tank + extra bypass)
% Valve return to tank/return line:
Q_return_valve = max(Q_AT,0) + max(Q_BT,0);  % [m^3/s]

% C_bypass ≈ 6.43e-13 m^3/(s*Pa)
C_bypass = 6.43e-13; %1.628161 * 0.6*1.1;
Q_bypass = C_bypass * max(P_P - P_R, 0);     % [m^3/s]

Q_return_total = Q_return_valve + Q_bypass;
Q_return_model_lpm   = 60000 * Q_return_total;

%% 11) Leakage indicator (trend)
Q_Leak_Total = 0.5*(abs(Q_PA) + abs(Q_PB) + abs(Q_AT) + abs(Q_BT)) ...
              - 0.5*abs(Q_A + Q_B);
Q_Leak_Total_lpm = Q_Leak_Total * 60e3;
end

== matlab function phdMain/Cylinder_Dynamics/Subsystem/Subsystem/MATLAB Function ==
  data: v input; F_statik output
function F_statik = fcn(v)
Fc = 18; 
Fs = 75; 
v_s = 0.016; 
C = 100; 

F_statik = Fc + (Fs - Fc)*exp(-(1*abs(v)./v_s)^2);
F_statik = F_statik * tanh(C*v);
